simulink model "AtcaEKFsRpZp"  (R2024b)
settings: Solver=FixedStepAuto  StartTime=0.0  StopTime=10.0  RelTol=1e-3
undefined symbols (not defined in the file): C1, C2, C3, C4, Ip_threshold, maxMirnovConfidence
settings Model: Creator=felipe  LastModifiedBy=felipe
settings OptimizationCC: PassReuseOutputArgsAs=Individual arguments  OptimizeBlockOrder=speed  DifferentSizesBufferReuse=on  EfficientTunableParamExpr=on
settings DebuggingCC: ParameterTunabilityLossMsg=error
settings HardwareCC: TargetBitPerLong=64  TargetBitPerPointer=64  TargetBitPerSizeT=64  TargetBitPerPtrDiffT=64  TargetLongLongMode=on  TargetIntDivRoundTo=Zero  TargetEndianess=LittleEndian  TargetWordSize=64  TargetHWDeviceType=MATLAB Host  ProdEqTarget=off
settings SFSimCC: MATLABDynamicMemAlloc=off
settings RTWCC: Description=Embedded Coder (host-based shared library target)  SystemTargetFile=ert_shrlib.tlc  TemplateMakefile=ert_default_tmf  RTWVerbose=off
settings RTWCC: CustomSourceCode=|
  | #define CONCAT(str1, str2, str3) CONCAT_(str1, str2, str3)
  | #define CONCAT_(str1, str2, str3) str1 ## str2 ## str3
  | #define GET_MMI_FUNC    CONCAT(MODEL  , _GetCAPImmi ,  )
  | #define RT_MODEL_STRUCT CONCAT(RT_MODEL_ , MODEL  , _T )
  | 
  | void* GET_MMI_FUNC(void* voidPtrToRealTimeStructure)
  | {
  | rtwCAPI_ModelMappingInfo* mmiPtr = &(rtmGetDataMapInfo( ( RT_MODEL_STRUCT * )(voidPtrToRealTimeStructure) ).mmi);
  | return (void*) mmiPtr;
  | }
settings CodeAppCC: GenerateComments=off  IgnoreCustomStorageClasses=off  OperatorAnnotations=on  SimulinkDataObjDesc=on  SFDataObjDesc=on  SimulinkBlockComments=off
settings STFCustomTargetCC: TargetLangStandard=C99 (ISO)  MultiwordLength=256  ParMdlRefBuildCompliant=on  CompOptLevelCompliant=on  IncludeMdlTerminateFcn=off  CombineOutputUpdateFcns=on  CombineSignalStateStructs=on  SuppressErrorStatus=on  ERTCustomFileBanners=on  SupportAbsoluteTime=off  CodeInterfacePackaging=Reusable function  SupportComplex=off  SupportContinuousTime=off  SupportNonInlinedSFcns=off  RemoveResetFunc=on  MATLABClassNameForMDSCustomization=Simulink.SoftwareTarget.ERTCustomization  ModelStepFunctionPrototypeControlCompliant=on  GenerateAllocFcn=on  UseToolchainInfoCompliant=on  SystemTargetFile=ert_shrlib.tlc
settings ERTTargetCC: TargetLangStandard=C99 (ISO)  ConcurrentExecutionCompliant=off  IncludeMdlTerminateFcn=off  CombineSignalStateStructs=on  SuppressErrorStatus=on  SupportAbsoluteTime=off  CodeInterfacePackaging=Reusable function  SupportComplex=off  CPPClassGenCompliant=off  GenerateAllocFcn=on  InlinedParameterPlacement=Hierarchical  RootIOFormat=Part of model data structure  RTWCAPIParams=on  RTWCAPIRootIO=on  ERTCustomFileTemplate=example_file_process.tlc

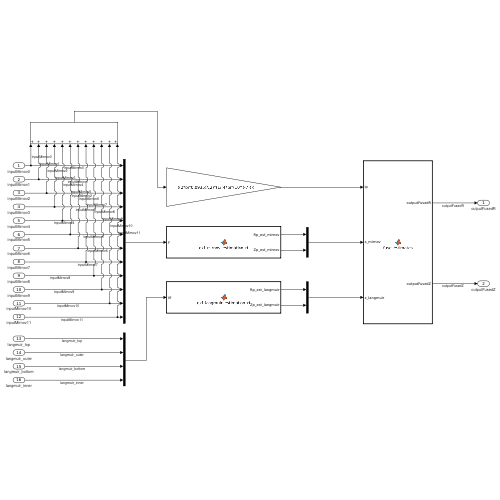
[thumbnail: Simulink's stored preview of the top-level diagram]
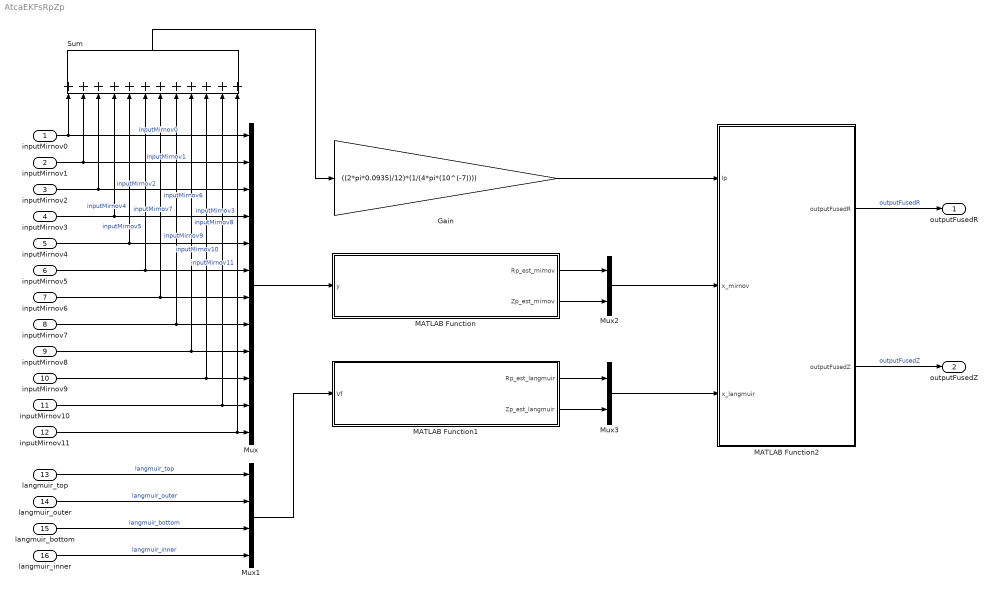
== system AtcaEKFsRpZp ==
  inputMirnov0 : Inport  OutDataTypeStr=single
  inputMirnov1 : Inport  Port=2  OutDataTypeStr=single
  inputMirnov2 : Inport  Port=3  OutDataTypeStr=single
  inputMirnov3 : Inport  Port=4  OutDataTypeStr=single
  inputMirnov4 : Inport  Port=5  OutDataTypeStr=single
  inputMirnov5 : Inport  Port=6  OutDataTypeStr=single
  inputMirnov6 : Inport  Port=7  OutDataTypeStr=single
  inputMirnov7 : Inport  Port=8  OutDataTypeStr=single
  inputMirnov8 : Inport  Port=9  OutDataTypeStr=single
  inputMirnov9 : Inport  Port=10  OutDataTypeStr=single
  inputMirnov10 : Inport  Port=11  OutDataTypeStr=single
  inputMirnov11 : Inport  Port=12  OutDataTypeStr=single
  langmuir_top : Inport  Port=13  OutDataTypeStr=single
  langmuir_outer : Inport  Port=14  OutDataTypeStr=single
  langmuir_bottom : Inport  Port=15  OutDataTypeStr=single
  langmuir_inner : Inport  Port=16  OutDataTypeStr=single
  Gain : Gain  Gain=((2*pi*0.0935)/12)*(1/(4*pi*(10^(-7))))  OutDataTypeStr=single
  MATLAB Function : MATLAB Function  TreatAsAtomicUnit=on
  MATLAB Function1 : MATLAB Function  TreatAsAtomicUnit=on
  MATLAB Function2 : MATLAB Function  TreatAsAtomicUnit=on
  Mux : Mux  Inputs=12
  Mux1 : Mux
  Mux2 : Mux  Inputs=2
  Mux3 : Mux  Inputs=2
  Sum : Sum  Inputs=++++++++++++  OutDataTypeStr=single  AccumDataTypeStr=single
  outputFusedR : Outport  OutDataTypeStr=single
  outputFusedZ : Outport  Port=2  OutDataTypeStr=single
  wires:
  langmuir_top/1 -> Mux1/1  "langmuir_top"
  langmuir_outer/1 -> Mux1/2  "langmuir_outer"
  langmuir_bottom/1 -> Mux1/3  "langmuir_bottom"
  langmuir_inner/1 -> Mux1/4  "langmuir_inner"
  inputMirnov0/1 -> Mux/1, Sum/1  "inputMirnov0"
  inputMirnov1/1 -> Mux/2, Sum/2  "inputMirnov1"
  inputMirnov2/1 -> Mux/3, Sum/3  "inputMirnov2"
  inputMirnov3/1 -> Mux/4, Sum/4  "inputMirnov3"
  inputMirnov4/1 -> Mux/5, Sum/5  "inputMirnov4"
  inputMirnov5/1 -> Mux/6, Sum/6  "inputMirnov5"
  inputMirnov6/1 -> Mux/7, Sum/7  "inputMirnov6"
  inputMirnov7/1 -> Mux/8, Sum/8  "inputMirnov7"
  inputMirnov8/1 -> Mux/9, Sum/9  "inputMirnov8"
  inputMirnov9/1 -> Mux/10, Sum/10  "inputMirnov9"
  inputMirnov10/1 -> Mux/11, Sum/11  "inputMirnov10"
  inputMirnov11/1 -> Mux/12, Sum/12  "inputMirnov11"
  Mux/1 -> MATLAB Function/1(y)
  Mux1/1 -> MATLAB Function1/1(Vf)
  MATLAB Function/1(Rp_est_mirnov) -> Mux2/1
  MATLAB Function/2(Zp_est_mirnov) -> Mux2/2
  MATLAB Function1/1(Rp_est_langmuir) -> Mux3/1
  MATLAB Function1/2(Zp_est_langmuir) -> Mux3/2
  Mux2/1 -> MATLAB Function2/2(x_mirnov)
  Mux3/1 -> MATLAB Function2/3(x_langmuir)
  MATLAB Function2/2(outputFusedZ) -> outputFusedZ/1  "outputFusedZ"
  MATLAB Function2/1(outputFusedR) -> outputFusedR/1  "outputFusedR"
  Sum/1 -> Gain/1
  Gain/1 -> MATLAB Function2/1(Ip)

== matlab function AtcaEKFsRpZp/MATLAB Function1 ==
  data: Vf input single size=[4 1]; Rp_est_langmuir output single; Zp_est_langmuir output single; C1 parameter single; C2 parameter single; C3 parameter single; C4 parameter single
function [Rp_est_langmuir, Zp_est_langmuir] = ekf_langmuir_estimation_rt(Vf, C1, C2, C3, C4)
    % Extended Kalman Filter for plasma position estimation using Langmuir probes
    %
    %   This function implements the update step of an Extended Kalman Filter (EKF)
    %   to estimate the radial (Rp) and vertical (Zp) positions of the plasma current
    %   centroid based on floating potential measurements from 4 Langmuir probes.
    %
    % Inputs:
    %   Vf - [4x1] vector with floating potentials (top; outer; bottom;
    %   inner) [V]
    %   
    % Outputs:
    %   Rp_est_langmuir - Estimated radial position of plasma [m]
    %   Zp_est_langmuir - Estimated vertical position of plasma [m]
    %   P_langmuir      - [2x2] Covariance matrix of the current state estimate

    persistent x P_int Q R

    if isempty(x)
        % Initial state: assume plasma is centered
        x = single([0.46; 0.0]); % [Rp; Zp]
    end

    if isempty(P_int)
        % Initial covariance matrix (uncertainty):
        % Rp: ±2.5 cm, Zp: ±2.5 cm
        P_sigma_pos = single(0.025);
        corr_pos = single(-0.0122743585580109); % Correlation between Rp and Zp
        
        P_int = single([P_sigma_pos^2, corr_pos * P_sigma_pos^2;
             corr_pos * P_sigma_pos^2, P_sigma_pos^2]);
    end

    if isempty(Q)
        % Process noise
        Q = single(diag([(0.020)^2, (0.010)^2]));
    end

    if isempty(R)
        % Measurement noise (floating potential variance)
        R = single(diag([(1.5)^2, (1.5)^2, (1.5)^2, (1.5)^2]));
    end

    % Prediction step (no state model used)
    x_pred = x;
    P_pred = P_int + Q;

    % Measurement function h(x) using Langmuir model
    y = Vf;  % Direct measurement from Langmuir probes
    y_pred = computeLangmuirPotentials(x_pred, C1, C2, C3, C4);  % Predicted Vf from current state estimate
    H_langmuir = jacobian_h(C1, C2, C3, C4);  % Jacobian matrix of h(x)

    % Kalman gain
    K_langmuir = P_pred * H_langmuir' / (H_langmuir * P_pred * H_langmuir' + R);

    % Update step
    x = x_pred + K_langmuir * (y - y_pred);
    P_int = (eye(2, 'single') - K_langmuir * H_langmuir) * P_pred;

    % Output
    Rp_est_langmuir = x(1);
    Zp_est_langmuir = x(2);
end

function Vf = computeLangmuirPotentials(x, C1, C2, C3, C4)
    % Computes the expected floating potentials based on plasma position
    % using a centered inverse of the Langmuir model.
    %
    % Inputs:
    %   x - [Rp; Zp] plasma position estimate
    % Outputs:
    %   Vf - [4x1] predicted floating potentials: [top; outer; bottom; inner]

    Rp = x(1);
    Zp = x(2);  % Ou Vp, se estiver usando tensão vertical em vez da posição

    % Coefficients from the Langmuir probe model
    [coef1, coef2, coef3, coef4] = langmuirCoefficients(C1, C2, C3, C4);

    % Calculate differences based on the inverse of the model
    delta_R = (Rp - coef2) / coef1;
    delta_Z = (Zp - coef4) / coef3;

    % Centered solution (mean of each pair is zero)
    Vf_outer  = single(0.5) * delta_R;
    Vf_inner  = single(-0.5) * delta_R;
    Vf_top    = single(0.5) * delta_Z;
    Vf_bottom = single(-0.5) * delta_Z;

    Vf = single([Vf_top; Vf_outer; Vf_bottom; Vf_inner]);
end

function H_langmuir = jacobian_h(C1, C2, C3, C4)
    % Jacobian matrix of h(x) = Vf with respect to x = [Rp; Zp]

    % Coefficients from the Langmuir probe model
    [coef1, ~, coef3, ~] = langmuirCoefficients(C1, C2, C3, C4);

    % Derivatives of each Vf component with respect to [Rp; Zp]
    dVf_top_dRp = single(0);
    dVf_top_dZp = single(0.5) / coef3;

    dVf_outer_dRp = single(0.5) / coef1;
    dVf_outer_dZp = single(0);

    dVf_bottom_dRp = single(0);
    dVf_bottom_dZp = single(-0.5) / coef3;

    dVf_inner_dRp = single(-0.5) / coef1;
    dVf_inner_dZp = single(0);

    % H_langmuir is a 4x2 matrix: one row per output, one column per state variable
    H_langmuir = single([
        dVf_top_dRp,    dVf_top_dZp;
        dVf_outer_dRp,  dVf_outer_dZp;
        dVf_bottom_dRp, dVf_bottom_dZp;
        dVf_inner_dRp,  dVf_inner_dZp
    ]);
end

function [coef1, coef2, coef3, coef4] = langmuirCoefficients(C1, C2, C3, C4)
    coef1 = C1; %C1 = 5.0954483801905011e-04;
    coef2 = C2; %C2 = 4.2525165579344343e-01;
    coef3 = C3; %C3 = -2.9966557416733034e-04;
    coef4 = C4; %C4 = -2.6182024607468400e-03;
end

== matlab function AtcaEKFsRpZp/MATLAB Function ==
  data: y input single size=[12 1]; Rp_est_mirnov output single; Zp_est_mirnov output single
function [Rp_est_mirnov, Zp_est_mirnov] = ekf_mirnov_estimation_rt(y)
    % Extended Kalman Filter for plasma position estimation using Mirnov coils
    %
    %   This function implements the update step of an Extended Kalman Filter (EKF)
    %   for estimating the radial (Rp) and vertical (Zp) positions of the plasma
    %   current centroid based on magnetic field measurements from 12 Mirnov coils.
    %
    % Inputs:
    %   y - [12x1] vector of magnetic field measurements from Mirnov coils [T]
    %
    % Outputs:
    %   Rp_est_mirnov - estimated radial position of plasma [m]
    %   Zp_est_mirnov - estimated vertical position of plasma [m]
    %   P_mirnov      - [2x2] Covariance matrix of the current state estimate

    persistent x P_int mirnov_pos Q R

    if isempty(x)
        % Initial state (assume centered plasma)
        x = single([0.46; 0.0]);  % Initial state: Rp = 0.46 m, Zp = 0.0 m
    end

    if isempty(P_int)
        % Initial covariance matrix (uncertainty):
        % Rp: ±2.5 cm, Zp: ±2.5 cm
        P_sigma_pos = single(0.025);
        corr_pos = single(0.4186145127102582); % Correlation between Rp and Zp

        P_int = single([ P_sigma_pos^2,  corr_pos * P_sigma_pos^2;
              corr_pos * P_sigma_pos^2,  P_sigma_pos^2 ]);
    end

    % Mirnov coil geometry initialization (static)
    N = 12;
    mirnov_radius = single(0.0935);
    R0 = single(0.46);
    mirnov_pos = zeros(N, 2, 'single');
    for i = 1:N
        angle_deg = mod(15 - (i-1)*30, 360);
        mirnov_pos(i, :) = single([R0 + mirnov_radius * cosd(angle_deg), mirnov_radius * sind(angle_deg)]);
    end
    
    if isempty(Q)
        % Process noise (model deviation):
        % Rp: ±1.5 cm, Zp: ±1.5 cm
        Q = single(diag([(0.015)^2, (0.015)^2]));
    end

    if isempty(R)
        % Measurement noise (sensor accuracy)
        R_diag = single((1e-3)^2 * ones(N, 1, 'single'));
        R_diag(3) = single((1.5e-2)^2);     % Coil 3 (extreme noise)
        R_diag(10) = single((7.5e-3)^2);    % Coil 10 (significant noise)
        R = single(diag(R_diag));
    end
    
    % Prediction step (no state model used)
    x_pred = x;
    P_pred = P_int + Q;

    % Update step (EKF)
    B_total = sum(y);  % Real-time constraint from measurements
    H_mirnov = jacobian_h(x_pred, mirnov_pos, B_total);
    y_pred = computeMirnovFields(x_pred, mirnov_pos, B_total);
    K_mirnov = P_pred * H_mirnov' / (H_mirnov * P_pred * H_mirnov' + R);
    x = x_pred + K_mirnov * (y - y_pred);
    P_int = (eye(2, 'single') - K_mirnov * H_mirnov) * P_pred;

    % Outputs
    Rp_est_mirnov = x(1);
    Zp_est_mirnov = x(2);
end

function H_mirnov = jacobian_h(x, mirnov_pos, B_total)
    eps = single(1e-4);
    n = length(x);
    m = size(mirnov_pos, 1);
    H_mirnov = zeros(m, n, 'single');
    for j = 1:n
        dx = zeros(n,1,'single');
        dx(j) = eps;
        H_mirnov(:,j) = (computeMirnovFields(x + dx, mirnov_pos, B_total) - computeMirnovFields(x - dx, mirnov_pos, B_total)) / (single(2)*eps);
    end
end

function B = computeMirnovFields(x, mirnov_pos, B_total)
    % Compute the expected magnetic field measurements (B_i) for the 12 Mirnov coils
    % given a predicted plasma current center [Rp, Zp] and total magnetic field B_total.

    % Geometry constants
    R0 = single(0.46);               % Major radius (m)
    a = single(0.085);               % Minor radius (m)
    delta_R = a^2 / (single(4) * R0);  % Geometrical correction term

    % Extract positions from mirnov_pos
    R = mirnov_pos(:, 1);
    Z = mirnov_pos(:, 2);
    N = length(R);
    
    Rp = x(1);
    Zp = x(2);

    % Build constraint matrix A
    A = zeros(3, N, 'single');
    A(1, :) = R' - Rp + delta_R;  % Horizontal constraint (Rp)
    A(2, :) = Z' - Zp;            % Vertical constraint (Zp)
    A(3, :) = ones(1, N, 'single');         % Sum(B_i) = B_total

    % Constraint vector
    c = single([0; 0; B_total]);

    % Solve for minimum-norm B satisfying A*B = c
    B = A' * ((A * A') \ c);
end

== matlab function AtcaEKFsRpZp/MATLAB Function2 ==
  data: Ip input; outputFusedR output; x_mirnov input single size=[2 1]; x_langmuir input single size=[2 1]; outputFusedZ output single; Ip_threshold parameter single; maxMirnovConfidence parameter single
function [outputFusedR, outputFusedZ] = fuse_estimates(Ip, x_mirnov, x_langmuir, Ip_threshold, maxMirnovConfidence)
    % Function to fuse two state estimates from independent EKFs (Mirnov and Langmuir)
    %
    %   This function fuses the estimated states [Rp; Zp] from two separate EKFs
    %   using a dynamic weighting scheme based on the plasma current. As |Ip| increases,
    %   more confidence is given to the magnetic (Mirnov) estimation..
    %
    % Inputs:
    %   Ip           - Plasma current [A]
    %   Ip_threshold - Reference plasma current [A] used to modulate the confidence
    %                  in the Mirnov-based estimation. As |Ip| approaches this value,
    %                  the fusion gives progressively more weight to the Mirnov EKF.
    %                  Below this threshold, Langmuir estimates dominate.
    %   maxMirnovConfidence - Maximum allowed confidence (weight) for the Mirnov-based
    %                        estimation during fusion. When |Ip| reaches |Ip_threshold|,
    %                        this value defines the highest fusion weight assigned
    %                        to the Mirnov estimate (range: 0 to 1.0).
    %   x_mirnov     - [2x1] state estimate from Mirnov EKF (Rp; Zp)
    %   x_langmuir   - [2x1] state estimate from Langmuir EKF (Rp; Zp)
    %
    % Outputs:
    %   outputFusedR - Fused estimate of Rp [m]
    %   outputFusedZ - Fused estimate of Zp [m]
    

    % Adaptive fusion based on normalized plasma current (alpha)
    % As |Ip| approaches Ip_threshold, more weight is given to Mirnov-based estimation
    
    % Compute fusion coefficient alpha (confidence in Mirnov)
    alpha = single(min(abs(Ip) / abs(Ip_threshold), 1)) * single(maxMirnovConfidence);  % Bound alpha between 0 and maxMirnovConfidence
    
    % Weighted fusion using alpha
    x_fused = alpha * x_mirnov + (single(1) - alpha) * x_langmuir;
    
    outputFusedR = x_fused(1);
    outputFusedZ = x_fused(2);
end
